simulink model "TP7_EJ6"  (R2020a)
settings: Solver=VariableStepAuto  StartTime=0.0  StopTime=20  RelTol=1e-3
values from neighbouring files (symbols this model uses):
  c1 = 50    [TP7_EJ3_matrices.m]    (also in TP7_EJ6_matrices.m = 2; TP7_EJ8.m = 2000)
  c2 = 50    [TP7_EJ3_matrices.m]    (also in TP7_EJ6_matrices.m = 3)
  k1 = 104    [TP7_EJ3_matrices.m]    (also in TP7_EJ6_matrices.m = 1; TP7_EJ8.m = 22000)
  k2 = k1*1.5    (= 156)    [TP7_EJ3_matrices.m]    (also in TP7_EJ6_matrices.m = 4; TP7_EJ8.m = 22000)
  m1 = 50    [TP7_EJ3_matrices.m]    (also in TP7_EJ6_matrices.m = 1; TP7_EJ8.m = 250)
  m2 = m1    (= 50)    [TP7_EJ3_matrices.m]    (also in TP7_EJ6_matrices.m = 1; TP7_EJ8.m = 25)
settings Model: Creator=Adriana  LastModifiedBy=Adriana

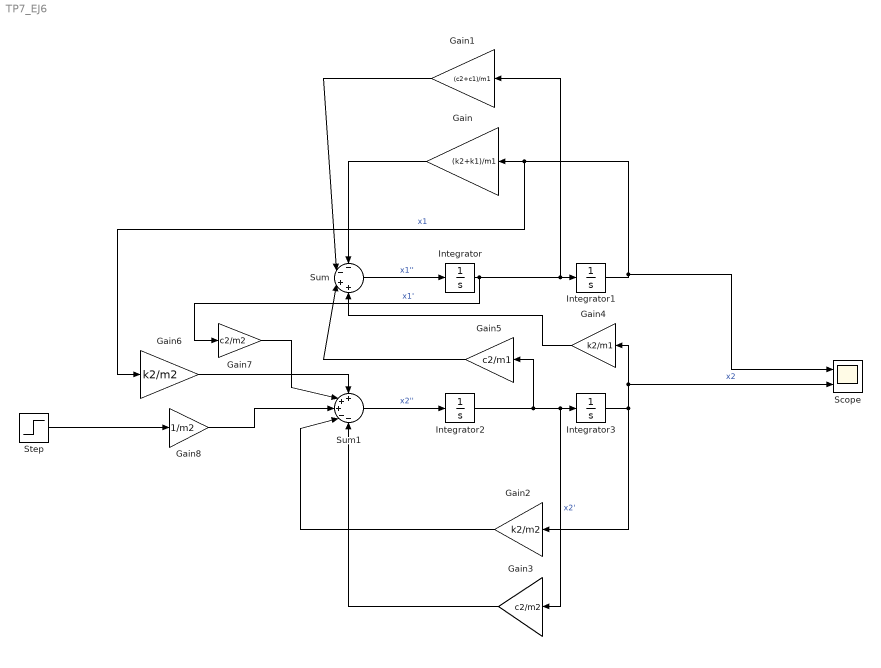
== system TP7_EJ6 ==
  Gain : Gain  Gain=(k2+k1)/m1
  Gain1 : Gain  Gain=(c2+c1)/m1
  Gain2 : Gain  Gain=k2/m2
  Gain3 : Gain  Gain=c2/m2
  Gain4 : Gain  Gain=k2/m1
  Gain5 : Gain  Gain=c2/m1
  Gain6 : Gain  Gain=k2/m2
  Gain7 : Gain  Gain=c2/m2
  Gain8 : Gain  Gain=1/m2
  Integrator{,1..3} (4 alike) : Integrator
  Scope : Scope  NumInputPorts=2
  Step : Step  SampleTime=0
  Sum : Sum  Inputs=--++
  Sum1 : Sum  Inputs=+++--
  wires:
  Sum/1 -> Integrator/1  "x1''"
  Integrator/1 -> Gain7/1, Gain1/1, Integrator1/1  "x1'"
  Integrator1/1 -> Scope/1, Gain/1, Gain6/1  "x1"
  Gain/1 -> Sum/1
  Gain1/1 -> Sum/2
  Sum1/1 -> Integrator2/1  "x2''"
  Integrator2/1 -> Gain5/1, Gain3/1, Integrator3/1  "x2'"
  Integrator3/1 -> Scope/2, Gain4/1, Gain2/1  "x2"
  Gain2/1 -> Sum1/4
  Gain5/1 -> Sum/3
  Gain4/1 -> Sum/4
  Gain3/1 -> Sum1/5
  Gain6/1 -> Sum1/1
  Gain7/1 -> Sum1/2
  Step/1 -> Gain8/1
  Gain8/1 -> Sum1/3
